simulink model "PPS_Scenario_006_cs"  (Simulink 7.6)
settings: Solver=ode5  SolverMode=SingleTasking  StartTime=0.0  StopTime=inf  FixedStep=1/100  RelTol=1e-3
PreLoadFcn:
  | check_NUTS_defined;
  | 
  | assignin('base',['model_closed_' bdroot],false);
  | 
  | addpath('../includes_PPS');
  | 
  | if exist('PPS_Model_sfun.mexw64')==3
  | delete PPS_Model_sfun.mexw64;
  | end
  | 
  | if exist('PPS_Model_sfun.mexw32') ==3
  | delete PPS_Model_sfun.mexw32;
  | end
  | 
  | switch version('-release')
  | case {'2010a', '2010b', '2011a'}
  | addpath('../includes_PPS/ML2010a');
  | case {'2011b', '2012a', '2012b'}
  | addpath('../includes_PPS/ML2011b');
  | otherwise
  | addpath('../includes_PPS/ML2011b');
  | end
InitFcn:
  | PreScanExperimentInitFcn(bdroot)
StopFcn:
  | PreScanExperimentStopFcn(bdroot)
undefined symbols (not defined in the file): DiscIntNeverNeededParam, InitImageOutputDir, x_ini_VRML, y_ini_VRML, z_ini_VRML
libraries: PreScanSimulinkLibrary x48, simulink x27, PreScanUsefulBlocks x20, simulink_extras x9, simulink_need_slupdate x1
(part 10 of 14)

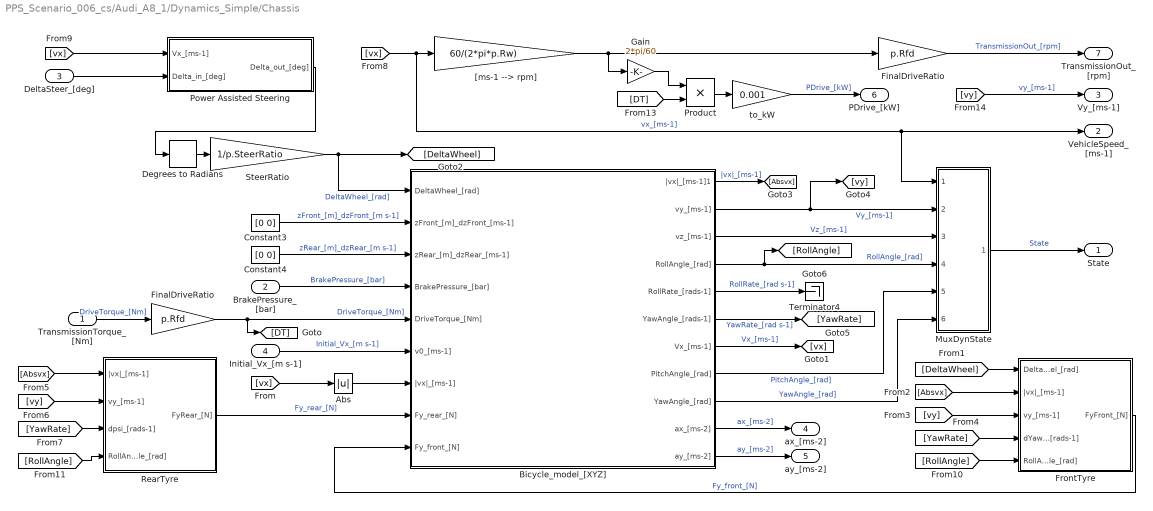
== system PPS_Scenario_006_cs/Audi_A8_1/Dynamics_Simple/Chassis ==
  TransmissionTorque_[Nm] : Inport
  BrakePressure_[bar] : Inport  Port=2
  DeltaSteer_[deg] : Inport  Port=3
  Initial_Vx_[m s-1] : Inport  Port=4
  Abs : Abs
  Bicycle_model_[XYZ] : Subsystem
      mask Display: image(imread('Bicycle_model.png'));
  Constant3 : Constant  Value=[0 0]
  Constant4 : Constant  Value=[0 0]
  Degrees to Radians : simulink_extras/Transformations/Degrees to Radians  SystemSampleTime=-1
  FinalDriveRatio : Gain  Gain=p.Rfd  SaturateOnIntegerOverflow=on  OutDataTypeStr=Inherit: Same as input  ParamDataTypeStr=Inherit: Same as input
  "FinalDriveRatio " : Gain  Gain=p.Rfd  SaturateOnIntegerOverflow=on  OutDataTypeStr=Inherit: Same as input  ParamDataTypeStr=Inherit: Same as input
  FrontTyre : Subsystem
      mask Display: image(imread('Tyre.png'));
  Gain : Gain  Gain=2*pi/60
  MuxDynState : Subsystem
  Power Assisted Steering : Subsystem
  Product : Product  RndMeth=Zero
  RearTyre : Subsystem
      mask Display: image(imread('Tyre.png'));
  SteerRatio : Gain  Gain=1/p.SteerRatio
  Terminator4 : Terminator
  "[ms-1 --> rpm]" : Gain  Gain=60/(2*pi*p.Rw)  SaturateOnIntegerOverflow=on  OutDataTypeStr=Inherit: Same as input  ParamDataTypeStr=Inherit: Same as input
  to_kW : Gain  Gain=0.001
  State : Outport
  VehicleSpeed_[ms-1] : Outport  Port=2
  Vy_[ms-1] : Outport  Port=3
  ax_[ms-2] : Outport  Port=4
  ay_[ms-2] : Outport  Port=5
  PDrive_[kW] : Outport  Port=6
  TransmissionOut_[rpm] : Outport  Port=7
  wires:
  [vy] -> Vy_[ms-1]/1  "vy_[ms-1]"
  to_kW/1 -> PDrive_[kW]/1  "PDrive_[kW]"
  Gain/1 -> Product/1
  Bicycle_model_[XYZ]/10(ax_[ms-2]) -> ax_[ms-2]/1  "ax_[ms-2]"
  Product/1 -> to_kW/1
  [DT] -> Product/2
  Bicycle_model_[XYZ]/11(ay_[ms-2]) -> ay_[ms-2]/1  "ay_[ms-2]"
  Abs/1 -> Bicycle_model_[XYZ]/7(|vx|_[ms-1])
  Degrees to Radians/1 -> SteerRatio/1
  [vx] -> Abs/1
  SteerRatio/1 -> [DeltaWheel], Bicycle_model_[XYZ]/1(DeltaWheel_[rad])  "DeltaWheel_[rad]"
  TransmissionTorque_[Nm]/1 -> "FinalDriveRatio "/1  "DriveTorque_[Nm]"
  RearTyre/1(FyRear_[N]) -> Bicycle_model_[XYZ]/8(Fy_rear_[N])  "Fy_rear_[N]"
  FrontTyre/1(FyFront_[N]) -> Bicycle_model_[XYZ]/9(Fy_front_[N])  "Fy_front_[N]"
  Bicycle_model_[XYZ]/1(|vx|_[ms-1]1) -> [Absvx]  "|vx|_[ms-1]"
  Bicycle_model_[XYZ]/2(vy_[ms-1]) -> [vy], MuxDynState/2(vy [ms-1])  "Vy_[ms-1]"
  Bicycle_model_[XYZ]/4(RollAngle_[rad]) -> MuxDynState/4(R [rad]), [RollAngle]  "RollAngle_[rad]"
  Bicycle_model_[XYZ]/6(YawAngle_[rads-1]) -> [YawRate]  "YawRate_[rad s-1]"
  Bicycle_model_[XYZ]/7(Vx_[ms-1]) -> [vx]  "Vx_[ms-1]"
  [DeltaWheel] -> FrontTyre/1(DeltaWheel_[rad])
  [Absvx] -> FrontTyre/2(|vx|_[ms-1])
  [vy] -> FrontTyre/3(vy_[ms-1])
  [YawRate] -> FrontTyre/4(dYawAngle_[rads-1])
  [Absvx] -> RearTyre/1(|vx|_[ms-1])
  [vy] -> RearTyre/2(vy_[ms-1])
  [YawRate] -> RearTyre/3(dpsi_[rads-1])
  Bicycle_model_[XYZ]/3(vz_[ms-1]) -> MuxDynState/3(vz [ms-1])  "Vz_[ms-1]"
  Bicycle_model_[XYZ]/8(PitchAngle_[rad]) -> MuxDynState/5(P [rad])  "PitchAngle_[rad]"
  Bicycle_model_[XYZ]/9(YawAngle_[rad]) -> MuxDynState/6(Y [rad])  "YawAngle_[rad]"
  "[ms-1 --> rpm]"/1 -> Gain/1, FinalDriveRatio/1
  FinalDriveRatio/1 -> TransmissionOut_[rpm]/1  "TransmissionOut_[rpm]"
  [vx] -> "[ms-1 --> rpm]"/1, VehicleSpeed_[ms-1]/1, MuxDynState/1(vx [ms-1])  "vx_[ms-1]"
  [vx] -> Power Assisted Steering/1(Vx_[ms-1])
  DeltaSteer_[deg]/1 -> Power Assisted Steering/2(Delta_in_[deg])
  Power Assisted Steering/1(Delta_out_[deg]) -> Degrees to Radians/1
  [RollAngle] -> FrontTyre/5(RollAngle_[rad])
  [RollAngle] -> RearTyre/4(RollAngle_[rad])
  Constant3/1 -> Bicycle_model_[XYZ]/2(zFront_[m]_dzFront_[ms-1])  "zFront_[m]_dzFront_[m s-1]"
  Constant4/1 -> Bicycle_model_[XYZ]/3(zRear_[m]_dzRear_[ms-1])  "zRear_[m]_dzRear_[m s-1]"
  BrakePressure_[bar]/1 -> Bicycle_model_[XYZ]/4(BrakePressure_[bar])  "BrakePressure_[bar]"
  "FinalDriveRatio "/1 -> Bicycle_model_[XYZ]/5(DriveTorque_[Nm]), [DT]  "DriveTorque_[Nm]"
  Initial_Vx_[m s-1]/1 -> Bicycle_model_[XYZ]/6(v0_[ms-1])  "Initial_Vx_[m s-1]"
  Bicycle_model_[XYZ]/5(RollRate_[rads-1]) -> Terminator4/1  "RollRate_[rad s-1]"
  MuxDynState/1(State) -> State/1  "State"

== system PPS_Scenario_006_cs/Audi_A8_1/Dynamics_Simple/Engine ==
  ImpellerTorque_[Nm] : Inport
  Throttle_[%] : Inport  Port=2
  Configurable Subsystem : Subsystem  BlockChoice=Discrete Rate Limiter  mask{ComputationMode=ComputationMode}
      mask prompts: ComputationMode "Compuation mode:"
      mask init:
      | SetComputationMode(gcb,ComputationMode);
      settings: AttributesFormatString=%<BlockChoice>  OpenFcn=BringToFront(gcb);  MemberBlocks=Discrete Rate Limiter,Rate Limiter
      settings: TemplateBlock=|
      | PreScanSimulinkLibrary/Configurable Subsystems/TransferFunction
      | Engine/Configurable
      | Subsystem
  Configurable Subsystem1 : Subsystem  BlockChoice=Discrete-Time Integrator  mask{ComputationMode=ComputationMode}
      mask prompts: ComputationMode "Computation mode:"
      mask init:
      | SetComputationMode(gcb,ComputationMode);
      settings: AttributesFormatString=%<BlockChoice>  OpenFcn=BringToFront(gcb);  MemberBlocks=Discrete-Time Integrator,Integrator
      settings: TemplateBlock=|
      | PreScanSimulinkLibrary/Configurable Subsystems/integral with initial condition and limts
      | for engine/Configurable
      | Subsystem
  EngineTorque : Lookup2D  RowIndex=p.thvec  ColumnIndex=p.nevec  Table=p.emap  InputSameDT=on
  Gain : Gain  Gain=2*pi/60
  Product : Product  RndMeth=Zero
  Sum : Sum  Inputs=-+  SaturateOnIntegerOverflow=on  InputSameDT=on  OutDataTypeStr=Inherit: Same as first input
  engine + impeller inertia : Gain  Gain=1/p.Iei  SaturateOnIntegerOverflow=on  OutDataTypeStr=Inherit: Same as input  ParamDataTypeStr=Inherit: Same as input
  to_kW : Gain  Gain=0.001
  nEngine_[rpm] : Outport  InitialOutput=0
  PEngine_[kW] : Outport  Port=2  InitialOutput=0
  wires:
  EngineTorque/1 -> Sum/2, Product/2
  engine + impeller inertia/1 -> Configurable Subsystem1/1(In1)
  Sum/1 -> engine + impeller inertia/1
  Configurable Subsystem1/1(Out1) -> nEngine_[rpm]/1, EngineTorque/2, Gain/1  "rpm"
  Throttle_[%]/1 -> Configurable Subsystem/1(In1)
  ImpellerTorque_[Nm]/1 -> Sum/1
  Configurable Subsystem/1(Out1) -> EngineTorque/1
  Product/1 -> to_kW/1
  Gain/1 -> Product/1
  to_kW/1 -> PEngine_[kW]/1

== system PPS_Scenario_006_cs/Audi_A8_1/Dynamics_Simple/Gear: Auto Manual ==
  note: 0; Auto = on // Manual =off
      | 1; Auto = off // Manual =on
  Auto_Manual : Inport
  Manual_Gear : Inport  Port=2
  Auto_Gear : Inport  Port=3
  If : If  IfExpression=u1 == 0
  If Action Subsystem : Subsystem  TreatAsAtomicUnit=on
  If Action Subsystem1 : Subsystem  TreatAsAtomicUnit=on
  Merge : Merge
  Gear : Outport
  wires:
  If Action Subsystem/1(Out1) -> Merge/1
  Auto_Gear/1 -> If Action Subsystem/1(In1)
  If/1 -> If Action Subsystem/Action
  Merge/1 -> Gear/1
  If Action Subsystem1/1(Out1) -> Merge/2
  Manual_Gear/1 -> If Action Subsystem1/1(In1)
  If/2 -> If Action Subsystem1/Action
  Auto_Manual/1 -> If/1

== system PPS_Scenario_006_cs/Audi_A8_1/Dynamics_Simple/ShiftLogic ==
  Throttle_[%] : Inport
  GearNr_[-] : Inport  Port=2
  Auto_GearShift : Inport  Port=3
  VehSpeed_[ms-1] : Inport  Port=4
  Add2 : Sum
  Data Type Conversion1 : DataTypeConversion  OutDataTypeStr=double
  Detect Increase1 : simulink/Logic and Bit Operations/Detect Increase  SystemSampleTime=-1  vinit=0.0
  Detect Increase : Subsystem
  Gear limitation : Saturate  UpperLimit=p.maxGear  LowerLimit=1
  Gear limitation while shifting : Saturate  UpperLimit=p.maxGear  LowerLimit=1
  GearNeutral : Constant  Value=0
  GearReverse : Constant  Value=-1
  "IC, gear = 1" : Memory  X0=1  InheritSampleTime=on
  If Action Neutral : Subsystem  TreatAsAtomicUnit=on
  If Action Normal : Subsystem  TreatAsAtomicUnit=on
  If Action Reverse : Subsystem  TreatAsAtomicUnit=on
  Memory : Memory  InheritSampleTime=on
  Merge : Merge  Inputs=3
  Relational Operator : RelationalOperator  OutDataTypeStr=boolean
  Relational Operator1 : RelationalOperator  Operator=<=  OutDataTypeStr=boolean
  Shift_Down time : simulink/Discrete/Integer Delay  NumDelays=p.ShiftDown_fac  InputProcessing=Inherited  vinit=0.0  samptime=-1
  Shift_Up time : simulink/Discrete/Integer Delay  NumDelays=p.ShiftUp_fac  InputProcessing=Inherited  vinit=0.0  samptime=-1
  Sum : Sum  Inputs=+-
  interp_down : Lookup2D  RowIndex=p.downth  ColumnIndex=[1:p.maxGear]  Table=p.downtab  LookUpMeth=Interpolation-Use End Values  InputSameDT=on
  interp_up : Lookup2D  RowIndex=p.upth  ColumnIndex=[1:p.maxGear]  Table=p.uptab  LookUpMeth=Interpolation-Use End Values  InputSameDT=on
  reverse/neutral/normal gear : If  IfExpression=u1 == 0  ElseIfExpressions=u1 < 0
  to_ms-1 : Gain  Gain=1/3.6
  "to_ms-1 " : Gain  Gain=1/3.6
  GearNr : Outport
  wires:
  Auto_GearShift/1 -> reverse/neutral/normal gear/1
  "IC, gear = 1"/1 -> If Action Normal/1(In1)
  Merge/1 -> GearNr/1
  If Action Reverse/1(Out1) -> Merge/2
  If Action Neutral/1(Out1) -> Merge/1
  If Action Normal/1(Out1) -> Merge/3
  reverse/neutral/normal gear/3 -> If Action Normal/Action
  reverse/neutral/normal gear/1 -> If Action Neutral/Action
  reverse/neutral/normal gear/2 -> If Action Reverse/Action
  GearReverse/1 -> If Action Reverse/1(In1)
  GearNeutral/1 -> If Action Neutral/1(In1)
  Shift_Down time/1 -> Sum/2
  Shift_Up time/1 -> Sum/1
  Detect Increase/1(Out1) -> Shift_Up time/1
  Data Type Conversion1/1 -> Shift_Down time/1
  Detect Increase1/1 -> Data Type Conversion1/1
  Sum/1 -> Add2/1
  Memory/1 -> Add2/2  "GearNr_[-]"
  Add2/1 -> Gear limitation while shifting/1
  Gear limitation while shifting/1 -> "IC, gear = 1"/1, Memory/1  "GearNr_[-]"
  Throttle_[%]/1 -> interp_down/1, interp_up/1
  Relational Operator/1 -> Detect Increase/2(In2)
  Relational Operator1/1 -> Detect Increase1/1
  interp_down/1 -> "to_ms-1 "/1
  VehSpeed_[ms-1]/1 -> Relational Operator/1, Relational Operator1/1
  interp_up/1 -> to_ms-1/1
  Gear limitation/1 -> interp_down/2, interp_up/2, Detect Increase/1(GearNr_[-])
  GearNr_[-]/1 -> Gear limitation/1
  to_ms-1/1 -> Relational Operator/2
  "to_ms-1 "/1 -> Relational Operator1/2

== system PPS_Scenario_006_cs/Audi_A8_1/Dynamics_Simple/Transmission ==
  nEngine_[rpm] : Inport
  GearNr_[-] : Inport  Port=2
  n_TransmissionOut_[rpm] : Inport  Port=3
  Torque_Converter : Subsystem
      mask Display: image(imread('TorqueConverter.png'));
  Transmission_Ratio : Subsystem
  Viscous coupling : Lookup  InputValues=[-5:0.1:5]*p.m/4  Table=p.m/4*tanh([-5:0.1:5])
  ImpellerTorque_[Nm] : Outport  InitialOutput=0
  TransmissionTorque_[Nm] : Outport  Port=2  InitialOutput=0
  wires:
  Torque_Converter/2(TurbineTorque_[Nm]) -> Viscous coupling/1  "Converter_Torque_[Nm]"
  Transmission_Ratio/2(nTransmissionIn_[rpm]) -> Torque_Converter/2(nTransmission_[rpm])
  nEngine_[rpm]/1 -> Torque_Converter/1(nEngine_[rpm])
  GearNr_[-]/1 -> Transmission_Ratio/2(GearNr_[-]), Torque_Converter/3(Gear nr)
  n_TransmissionOut_[rpm]/1 -> Transmission_Ratio/3(nTransmissionOut_[rpm])
  Torque_Converter/1(ImpellerTorque_[Nm]) -> ImpellerTorque_[Nm]/1
  Transmission_Ratio/1(tTransmissionOut_[Nm]) -> TransmissionTorque_[Nm]/1
  Viscous coupling/1 -> Transmission_Ratio/1(tTransmissionIn_[Nm])

== system PPS_Scenario_006_cs/Audi_A8_1/PathFollower_1/CTRL REFERENCES ==
  note: REFERENCE POSITION BASED POSITION CTRL
  Pos x,y,Y [m,m,rad] : Inport
  Position Preview Distance [m] : Inport  Port=2
  TrajOffset [m,m,rad] : Inport  Port=3
  ActorOffset_Left(+) / Right(-)_[m] : Inport  Port=4
  Calculate Preview Point (pvp) by extrapolating current Vehicle Position (p0) with Preview Distance and Vehicle Orientation : Subsystem
  Find Reference Point (pref)  on Trajectory closest  to PreView Point (pvp) : M-S-Function  FunctionName=msfcn_find_closest_trajectory_points  Parameters=[Traj_x Traj_y]
      mask Display:
      | port_label('input', 1, 'pvp')
      | port_label('input', 2, 'TrajOffset_x_y_Y')
      | port_label('input', 3, 'ActorOffset_Left+/Right-')
      | port_label('input', 4, 'p0')
      | port_label('output', 1, 'pref')
  Find Reference Point (pref0)  on Trajectory closest  to P0 Point (p0) : M-S-Function  FunctionName=msfcn_find_closest_trajectory_points0  Parameters=[Traj_x Traj_y]
      mask Display:
      | port_label('input', 1, 'pvp')
      | port_label('input', 2, 'TrajOffset_x_y_Y')
      | port_label('input', 3, 'ActorOffset_Left+/Right-')
      | port_label('input', 4, 'p0')
      | port_label('output', 1, 'pref_0')
      | port_label('output', 2, 'Actor/Traj_distance')
      | port_label('output', 3, 'Actor/Traj_angle')
  Mux1 : Mux  Inputs=2
  Selector1 : Selector  InputPortWidth=3  IndexOptions=Index vector (dialog)  Indices=[1 2]  OutputSizes=1
  Terminator : Terminator
  pvp  [m,m] : Outport
  pref_pvp [m,m] : Outport  Port=2
  pref_0 [m,m] : Outport  Port=3
  Actor/Traj_distance [m] : Outport  Port=4
  Actor/Traj_angle [deg] : Outport  Port=5
  wires:
  Mux1/1 -> pvp  [m,m]/1, Find Reference Point (pref)  on Trajectory closest  to PreView Point (pvp)/1, Find Reference Point (pref0)  on Trajectory closest  to P0 Point (p0)/1
  Pos x,y,Y [m,m,rad]/1 -> Calculate Preview Point (pvp) by extrapolating current Vehicle Position (p0) with Preview Distance and Vehicle Orientation/2(x,y,Y Demux [m,m,rad]), Find Reference Point (pref0)  on Trajectory closest  to P0 Point (p0)/4, Selector1/1
  Calculate Preview Point (pvp) by extrapolating current Vehicle Position (p0) with Preview Distance and Vehicle Orientation/1(x_glob_PVD) -> Mux1/1
  Calculate Preview Point (pvp) by extrapolating current Vehicle Position (p0) with Preview Distance and Vehicle Orientation/3(Y [rad]) -> Terminator/1
  Position Preview Distance [m]/1 -> Calculate Preview Point (pvp) by extrapolating current Vehicle Position (p0) with Preview Distance and Vehicle Orientation/1(Preview Distance)
  Find Reference Point (pref)  on Trajectory closest  to PreView Point (pvp)/1 -> pref_pvp [m,m]/1
  Find Reference Point (pref0)  on Trajectory closest  to P0 Point (p0)/1 -> pref_0 [m,m]/1
  Calculate Preview Point (pvp) by extrapolating current Vehicle Position (p0) with Preview Distance and Vehicle Orientation/2(y_glob_PVD) -> Mux1/2
  TrajOffset [m,m,rad]/1 -> Find Reference Point (pref)  on Trajectory closest  to PreView Point (pvp)/2, Find Reference Point (pref0)  on Trajectory closest  to P0 Point (p0)/2  "L6"
  ActorOffset_Left(+) / Right(-)_[m]/1 -> Find Reference Point (pref)  on Trajectory closest  to PreView Point (pvp)/3, Find Reference Point (pref0)  on Trajectory closest  to P0 Point (p0)/3
  Selector1/1 -> Find Reference Point (pref)  on Trajectory closest  to PreView Point (pvp)/4
  Find Reference Point (pref0)  on Trajectory closest  to P0 Point (p0)/2 -> Actor/Traj_distance [m]/1
  Find Reference Point (pref0)  on Trajectory closest  to P0 Point (p0)/3 -> Actor/Traj_angle [deg]/1

== system PPS_Scenario_006_cs/Audi_A8_1/PathFollower_1/Calculate shifted p0 wrt COG ==
  position x,y,Y [m,m,deg] : Inport
  Constant1 : Constant  Value=XShifting_wrt_COG
  Degrees to Radians : simulink_extras/Transformations/Degrees to Radians  SystemSampleTime=-1
  Demux1 : Demux  Outputs=3
  Fcn : Fcn  Expr=u(2)*cos(u(1))
  Fcn1 : Fcn  Expr=u(2)*sin(u(1))
  Mux1 : Mux  Inputs=3
  Mux2 : Mux  Inputs=2
  Sum : Sum  Inputs=|++
  Sum1 : Sum  Inputs=|++
  position x,y,Y [m,m,rad] : Outport
  wires:
  Sum/1 -> Mux1/1
  Sum1/1 -> Mux1/2
  Demux1/1 -> Sum/1
  Demux1/3 -> Degrees to Radians/1
  Degrees to Radians/1 -> Mux2/1, Mux1/3
  Mux2/1 -> Fcn/1, Fcn1/1
  Fcn/1 -> Sum/2
  Fcn1/1 -> Sum1/2
  Demux1/2 -> Sum1/1
  position x,y,Y [m,m,deg]/1 -> Demux1/1
  Mux1/1 -> position x,y,Y [m,m,rad]/1
  Constant1/1 -> Mux2/2

== system PPS_Scenario_006_cs/Audi_A8_1/PathFollower_1/DELTA CTRL ==
  note: POSITION BASED STEERWHEEL CONTROL
  p0 : Inport
  pvp : Inport  Port=2
  pref_pvp : Inport  Port=3
  pref0 : Inport  Port=4
  Calculate  preview angle : M-S-Function  FunctionName=msfcn_preview_angle_and_distance
      mask Display:
      | port_label('input', 2, 'pref [m,m]')
      | port_label('input', 3, 'p0 [m,m]')
      | port_label('input', 1, 'pvp [m,m]')
      | 
      | port_label('output', 1, 'angle [rad]')
  Divide2 : Product
  Divide4 : Product
  Error check : Subsystem
  Goto Tag Visibility : GotoTagVisibility  GotoTag=pref0
  Goto Tag Visibility1 : GotoTagVisibility  GotoTag=p0
  Radians to Degrees1 : simulink_extras/Transformations/Radians to Degrees  SystemSampleTime=-1
  Selector2 : Selector  InputPortWidth=3  IndexOptions=Index vector (dialog)  Indices=[1 2]  OutputSizes=1
  Steering angle  velocity dependent : Lookup  InputValues=[0 18 40 60 70 80 90 100 110]  Table=[16.5 16.5 28 44.5 55 60.5 60.5 60.5 60.5]
  Steering angle preview  distance dependent : Lookup  InputValues=[0 1 4 5 6 7 8 9 10 11 20 21]  Table=[1.5 1.5 1 1 1 1 1 1 0.9 0.9 0.8 0.8]
  These limits are  the vehicle maximum  steering wheel angle : Saturate  UpperLimit=720  LowerLimit=-720
  TunableSteering Gain : Gain  Gain=TunableSteeringGain
  sign1 : Gain  Gain=3.6
  delta_steerwheel [deg] : Outport
  tag scope: p0=scoped, pref0=scoped
  wires:
  Calculate  preview angle/1 -> Radians to Degrees1/1
  Selector2/1 -> Calculate  preview angle/3
  p0/1 -> Selector2/1, [p0]
  pvp/1 -> Calculate  preview angle/1
  pref_pvp/1 -> Calculate  preview angle/2
  Radians to Degrees1/1 -> Divide2/2
  These limits are  the vehicle maximum  steering wheel angle/1 -> delta_steerwheel [deg]/1
  pref0/1 -> [pref0]
  sign1/1 -> Steering angle  velocity dependent/1
  [v_actual] -> sign1/1
  Steering angle  velocity dependent/1 -> Divide2/1
  Divide4/1 -> TunableSteering Gain/1
  Divide2/1 -> Divide4/1
  Steering angle preview  distance dependent/1 -> Divide4/2
  [PreviewDistance] -> Steering angle preview  distance dependent/1
  TunableSteering Gain/1 -> These limits are  the vehicle maximum  steering wheel angle/1

== system PPS_Scenario_006_cs/Audi_A8_1/PathFollower_1/THROTTLE CTRL ==
  v_actual [m/s] : Inport
  Desired Velocity [m/s] : Inport  Port=2
  Initial Velocity [m/s] : Inport  Port=3
  Demux : Demux  Outputs=3
  GearNormal : Constant
  "GearNormal " : Constant
  If Desired Velocity = 0 : Subsystem  TreatAsAtomicUnit=on
  If Desired Velocity ~= 0 : Subsystem  TreatAsAtomicUnit=on
  Merge : Merge
  Mux : Mux  Inputs=3
  Mux2 : Mux  Inputs=3
  Sum4 : Sum  Inputs=|+-
  if : If  IfExpression=u1 == 0
  throttle [%] : Outport
  brake pressure [bar] : Outport  Port=2
  v0 [m/s] : Outport  Port=3
  Auto_GearShift : Outport  Port=4
  wires:
  v_actual [m/s]/1 -> Sum4/2
  If Desired Velocity ~= 0/3(Auto_GearShift) -> Mux2/3
  If Desired Velocity ~= 0/2(brake pressure [bar]) -> Mux2/2
  If Desired Velocity ~= 0/1(throttle [%]) -> Mux2/1
  if/1 -> If Desired Velocity = 0/Action
  if/2 -> If Desired Velocity ~= 0/Action
  If Desired Velocity = 0/3(Auto_GearShift) -> Mux/3
  "GearNormal "/1 -> If Desired Velocity ~= 0/1(In1)
  Demux/3 -> Auto_GearShift/1
  Demux/2 -> brake pressure [bar]/1
  Demux/1 -> throttle [%]/1
  Mux/1 -> Merge/1
  Mux2/1 -> Merge/2
  If Desired Velocity = 0/2(brake pressure [bar]) -> Mux/2
  If Desired Velocity = 0/1(throttle [%]) -> Mux/1
  Merge/1 -> Demux/1
  GearNormal/1 -> If Desired Velocity = 0/1(In1)
  Initial Velocity [m/s]/1 -> v0 [m/s]/1
  Desired Velocity [m/s]/1 -> Sum4/1, if/1
  Sum4/1 -> If Desired Velocity ~= 0/2(Desired Velocity [m/s])

== system PPS_Scenario_006_cs/Audi_A8_1/SELF_Demux/compas converter ==
  rotz [rad] : Inport
  cart2compas : Subsystem
  rad2deg : Gain  Gain=180/pi
  heading [deg] : Outport
  wires:
  cart2compas/1(heading [deg]) -> heading [deg]/1
  rotz [rad]/1 -> rad2deg/1
  rad2deg/1 -> cart2compas/1(Angle [deg])

== system PPS_Scenario_006_cs/Audi_A8_1/Trajectories/Car_trajectory_1 ==
  From Workspace : FromWorkspace  VariableName=trajectory  SampleTime=TimeStep  OutputAfterFinalValue=Holding final value
  From Workspace1 : FromWorkspace  VariableName=trajectory  SampleTime=TimeStep  OutputAfterFinalValue=Setting to zero
  Mux : Mux  Inputs=2
  Selector1 : Selector  InputPortWidth=24  IndexOptions=Index vector (dialog)  Indices=[7:18]  OutputSizes=1
  Selector9 : Selector  InputPortWidth=24  IndexOptions=Index vector (dialog)  Indices=[1:6]  OutputSizes=1
  trajectory : Outport
  wires:
  Selector1/1 -> Mux/2
  Selector9/1 -> Mux/1
  Mux/1 -> trajectory/1
  From Workspace1/1 -> Selector1/1
  From Workspace/1 -> Selector9/1

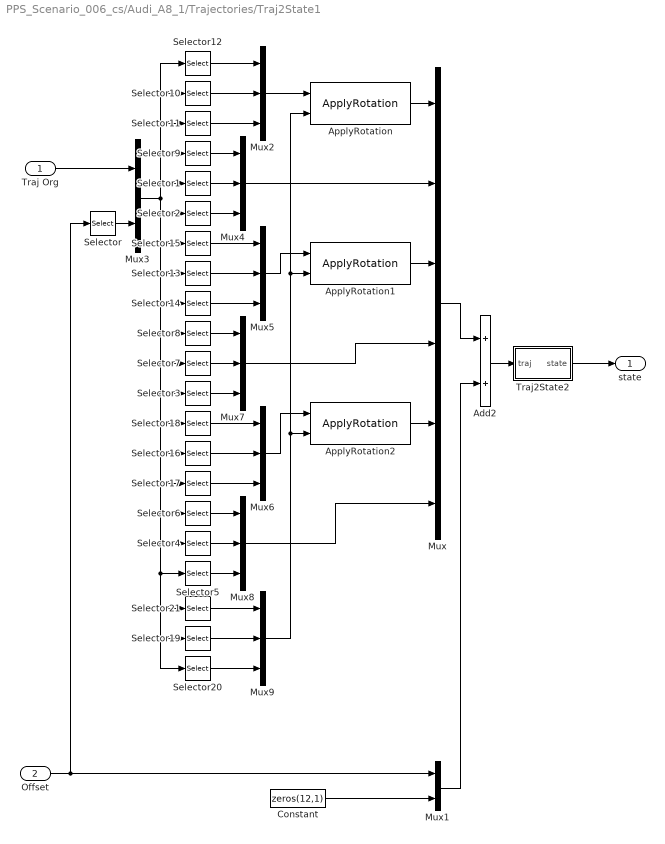
== system PPS_Scenario_006_cs/Audi_A8_1/Trajectories/Traj2State1 ==
  Traj Org : Inport
  Offset : Inport  Port=2
  Add2 : Sum
  ApplyRotation : PreScanSimulinkLibrary/ApplyRotation  SystemSampleTime=-1
  ApplyRotation1 : PreScanSimulinkLibrary/ApplyRotation  SystemSampleTime=-1
  ApplyRotation2 : PreScanSimulinkLibrary/ApplyRotation  SystemSampleTime=-1
  Constant : Constant  Value=zeros(12,1)
  Mux : Mux  Inputs=6
  Mux1 : Mux  Inputs=2
  Mux{2,4..9} (7 alike) : Mux  Inputs=3
  Mux3 : Mux  Inputs=2
  Selector : Selector  InputPortWidth=6  IndexOptions=Index vector (dialog)  Indices=[4 5 6]  OutputSizes=1
  Selector1 : Selector  InputPortWidth=21  IndexOptions=Index vector (dialog)  Indices=[5]  OutputSizes=1
  Selector10 : Selector  InputPortWidth=21  IndexOptions=Index vector (dialog)  Indices=[2]  OutputSizes=1
  Selector11 : Selector  InputPortWidth=21  IndexOptions=Index vector (dialog)  Indices=[3]  OutputSizes=1
  Selector12 : Selector  InputPortWidth=21  IndexOptions=Index vector (dialog)  Indices=[1]  OutputSizes=1
  Selector13 : Selector  InputPortWidth=21  IndexOptions=Index vector (dialog)  Indices=[8]  OutputSizes=1
  Selector14 : Selector  InputPortWidth=21  IndexOptions=Index vector (dialog)  Indices=[9]  OutputSizes=1
  Selector15 : Selector  InputPortWidth=21  IndexOptions=Index vector (dialog)  Indices=[7]  OutputSizes=1
  Selector16 : Selector  InputPortWidth=21  IndexOptions=Index vector (dialog)  Indices=[14]  OutputSizes=1
  Selector17 : Selector  InputPortWidth=21  IndexOptions=Index vector (dialog)  Indices=[15]  OutputSizes=1
  Selector18 : Selector  InputPortWidth=21  IndexOptions=Index vector (dialog)  Indices=[13]  OutputSizes=1
  Selector19 : Selector  InputPortWidth=21  IndexOptions=Index vector (dialog)  Indices=[20]  OutputSizes=1
  Selector2 : Selector  InputPortWidth=21  IndexOptions=Index vector (dialog)  Indices=[6]  OutputSizes=1
  Selector20 : Selector  InputPortWidth=21  IndexOptions=Index vector (dialog)  Indices=[21]  OutputSizes=1
  Selector21 : Selector  InputPortWidth=21  IndexOptions=Index vector (dialog)  Indices=[19]  OutputSizes=1
  Selector3 : Selector  InputPortWidth=21  IndexOptions=Index vector (dialog)  Indices=[12]  OutputSizes=1
  Selector4 : Selector  InputPortWidth=21  IndexOptions=Index vector (dialog)  Indices=[17]  OutputSizes=1
  Selector5 : Selector  InputPortWidth=21  IndexOptions=Index vector (dialog)  Indices=[18]  OutputSizes=1
  Selector6 : Selector  InputPortWidth=21  IndexOptions=Index vector (dialog)  Indices=[16]  OutputSizes=1
  Selector7 : Selector  InputPortWidth=21  IndexOptions=Index vector (dialog)  Indices=[11]  OutputSizes=1
  Selector8 : Selector  InputPortWidth=21  IndexOptions=Index vector (dialog)  Indices=[10]  OutputSizes=1
  Selector9 : Selector  InputPortWidth=21  IndexOptions=Index vector (dialog)  Indices=[4]  OutputSizes=1
  Traj2State2 : Subsystem
  state : Outport
  wires:
  Mux9/1 -> ApplyRotation2/2, ApplyRotation1/2, ApplyRotation/2
  Selector20/1 -> Mux9/3
  Selector19/1 -> Mux9/2
  Selector21/1 -> Mux9/1
  Selector5/1 -> Mux8/3
  Selector4/1 -> Mux8/2
  Selector6/1 -> Mux8/1
  Mux8/1 -> Mux/6
  Mux6/1 -> ApplyRotation2/1
  Mux7/1 -> Mux/4
  ApplyRotation2/1 -> Mux/5
  Selector3/1 -> Mux7/3
  Selector7/1 -> Mux7/2
  Selector8/1 -> Mux7/1
  Mux4/1 -> Mux/2
  Mux5/1 -> ApplyRotation1/1
  ApplyRotation1/1 -> Mux/3
  Mux2/1 -> ApplyRotation/1
  ApplyRotation/1 -> Mux/1
  Selector2/1 -> Mux4/3
  Selector1/1 -> Mux4/2
  Selector9/1 -> Mux4/1
  Selector17/1 -> Mux6/3
  Selector16/1 -> Mux6/2
  Selector18/1 -> Mux6/1
  Selector14/1 -> Mux5/3
  Selector13/1 -> Mux5/2
  Selector15/1 -> Mux5/1
  Selector11/1 -> Mux2/3
  Selector10/1 -> Mux2/2
  Selector12/1 -> Mux2/1
  Mux3/1 -> Selector8/1, Selector7/1, Selector3/1, Selector18/1, Selector16/1, Selector17/1, Selector6/1, Selector20/1, Selector19/1, Selector21/1, Selector5/1, Selector4/1, Selector14/1, Selector13/1, Selector15/1, Selector2/1, Selector1/1, Selector9/1, Selector12/1, Selector10/1, Selector11/1
  Mux1/1 -> Add2/2
  Constant/1 -> Mux1/2
  Add2/1 -> Traj2State2/1(traj)
  Selector/1 -> Mux3/2
  Traj Org/1 -> Mux3/1
  Offset/1 -> Mux1/1, Selector/1
  Mux/1 -> Add2/1
  Traj2State2/1(state) -> state/1

== system PPS_Scenario_006_cs/BMW_X5_1/Dynamics_Empty/MuxState ==
  note: mode: Dynamics
  note: mode: Positioning
  note: mode: Dynamics
      | VelVEHICLE
      | wrt VEH
  note: AnglesVEHICLE
      | wrtGLOB
  note: For state mode 'Dynamic' positions
      | are not taken into account, as they
      | are computed by integrating velocity.
      | Click annotation for Help.
  x [m] : Inport  SampleTime=TimeStep
  y [m] : Inport  Port=2  SampleTime=TimeStep
  z [m] : Inport  Port=3  SampleTime=TimeStep
  dx [m/s] : Inport  Port=4  SampleTime=TimeStep
  dy [m/s] : Inport  Port=5  SampleTime=TimeStep
  dz [m/s] : Inport  Port=6  SampleTime=TimeStep
  R [rad] : Inport  Port=7  SampleTime=TimeStep
  P [rad] : Inport  Port=8  SampleTime=TimeStep
  Y [rad] : Inport  Port=9  SampleTime=TimeStep
  Constant : Constant  DisableCoverage=on  Value=positioningmode
  Discrete-Time Integrator : DiscreteIntegrator  SampleTime=TimeStep  ICPrevOutput=DiscIntNeverNeededParam  ICPrevScaledInput=DiscIntNeverNeededParam
  Ground : Ground
  Ground1 : Ground
  Mux1 : Mux  Inputs=[3 3]
  Mux2 : Mux  Inputs=3
  Mux3 : Mux  Inputs=3
  Mux4 : Mux  Inputs=3
  Mux5 : Mux  Inputs=[3 3]
  Mux6 : Mux  Inputs=[6 3]
  Switch : Switch  Threshold=0.5
  Transformation_BODY2GLOBAL : PreScanSimulinkLibrary/Simple_Vehicle_Dynamics/Chassis/MuxDynState/Transformation_BODY2GLOBAL  SystemSampleTime=-1
  mux3 : Mux  Inputs=3
  state : Outport
  wires:
  Constant/1 -> Switch/2
  Mux6/1 -> state/1
  Mux4/1 -> Mux1/1
  Mux5/1 -> Switch/3
  Mux1/1 -> Switch/1
  Switch/1 -> Mux6/1  "PosVeh wrt  GLOB"
  P [rad]/1 -> Mux3/2
  R [rad]/1 -> Mux3/1
  dz [m/s]/1 -> Mux2/3
  dy [m/s]/1 -> Mux2/2
  dx [m/s]/1 -> Mux2/1
  z [m]/1 -> Mux4/3
  y [m]/1 -> Mux4/2
  x [m]/1 -> Mux4/1
  Ground1/1 -> mux3/2  "pitch"
  Y [rad]/1 -> mux3/3, Mux3/3  "yaw"
  Mux3/1 -> Mux6/2
  Transformation_BODY2GLOBAL/1 -> Discrete-Time Integrator/1, Mux5/2  "VelVEH wrt  GLOB"
  mux3/1 -> Transformation_BODY2GLOBAL/2
  Ground/1 -> mux3/1  "roll"
  Mux2/1 -> Mux1/2, Transformation_BODY2GLOBAL/1
  Discrete-Time Integrator/1 -> Mux5/1  "PosVEH wrt  GLOB"

== system PPS_Scenario_006_cs/BMW_X5_1/SELF_Demux/compas converter ==
  rotz [rad] : Inport
  cart2compas : Subsystem
  rad2deg : Gain  Gain=180/pi
  heading [deg] : Outport
  wires:
  cart2compas/1(heading [deg]) -> heading [deg]/1
  rotz [rad]/1 -> rad2deg/1
  rad2deg/1 -> cart2compas/1(Angle [deg])

== system PPS_Scenario_006_cs/BMW_X5_2/Dynamics_Empty/MuxState ==
  note: mode: Dynamics
  note: mode: Positioning
  note: mode: Dynamics
      | VelVEHICLE
      | wrt VEH
  note: AnglesVEHICLE
      | wrtGLOB
  note: For state mode 'Dynamic' positions
      | are not taken into account, as they
      | are computed by integrating velocity.
      | Click annotation for Help.
  x [m] : Inport  SampleTime=TimeStep
  y [m] : Inport  Port=2  SampleTime=TimeStep
  z [m] : Inport  Port=3  SampleTime=TimeStep
  dx [m/s] : Inport  Port=4  SampleTime=TimeStep
  dy [m/s] : Inport  Port=5  SampleTime=TimeStep
  dz [m/s] : Inport  Port=6  SampleTime=TimeStep
  R [rad] : Inport  Port=7  SampleTime=TimeStep
  P [rad] : Inport  Port=8  SampleTime=TimeStep
  Y [rad] : Inport  Port=9  SampleTime=TimeStep
  Constant : Constant  DisableCoverage=on  Value=positioningmode
  Discrete-Time Integrator : DiscreteIntegrator  SampleTime=TimeStep  ICPrevOutput=DiscIntNeverNeededParam  ICPrevScaledInput=DiscIntNeverNeededParam
  Ground : Ground
  Ground1 : Ground
  Mux1 : Mux  Inputs=[3 3]
  Mux2 : Mux  Inputs=3
  Mux3 : Mux  Inputs=3
  Mux4 : Mux  Inputs=3
  Mux5 : Mux  Inputs=[3 3]
  Mux6 : Mux  Inputs=[6 3]
  Switch : Switch  Threshold=0.5
  Transformation_BODY2GLOBAL : PreScanSimulinkLibrary/Simple_Vehicle_Dynamics/Chassis/MuxDynState/Transformation_BODY2GLOBAL  SystemSampleTime=-1
  mux3 : Mux  Inputs=3
  state : Outport
  wires:
  Constant/1 -> Switch/2
  Mux6/1 -> state/1
  Mux4/1 -> Mux1/1
  Mux5/1 -> Switch/3
  Mux1/1 -> Switch/1
  Switch/1 -> Mux6/1  "PosVeh wrt  GLOB"
  P [rad]/1 -> Mux3/2
  R [rad]/1 -> Mux3/1
  dz [m/s]/1 -> Mux2/3
  dy [m/s]/1 -> Mux2/2
  dx [m/s]/1 -> Mux2/1
  z [m]/1 -> Mux4/3
  y [m]/1 -> Mux4/2
  x [m]/1 -> Mux4/1
  Ground1/1 -> mux3/2  "pitch"
  Y [rad]/1 -> mux3/3, Mux3/3  "yaw"
  Mux3/1 -> Mux6/2
  Transformation_BODY2GLOBAL/1 -> Discrete-Time Integrator/1, Mux5/2  "VelVEH wrt  GLOB"
  mux3/1 -> Transformation_BODY2GLOBAL/2
  Ground/1 -> mux3/1  "roll"
  Mux2/1 -> Mux1/2, Transformation_BODY2GLOBAL/1
  Discrete-Time Integrator/1 -> Mux5/1  "PosVEH wrt  GLOB"

== system PPS_Scenario_006_cs/BMW_X5_2/SELF_Demux/compas converter ==
  rotz [rad] : Inport
  cart2compas : Subsystem
  rad2deg : Gain  Gain=180/pi
  heading [deg] : Outport
  wires:
  cart2compas/1(heading [deg]) -> heading [deg]/1
  rotz [rad]/1 -> rad2deg/1
  rad2deg/1 -> cart2compas/1(Angle [deg])

== system PPS_Scenario_006_cs/BMW_Z3_1/Dynamics_Empty/MuxState ==
  note: mode: Dynamics
  note: mode: Positioning
  note: mode: Dynamics
      | VelVEHICLE
      | wrt VEH
  note: AnglesVEHICLE
      | wrtGLOB
  note: For state mode 'Dynamic' positions
      | are not taken into account, as they
      | are computed by integrating velocity.
      | Click annotation for Help.
  x [m] : Inport  SampleTime=TimeStep
  y [m] : Inport  Port=2  SampleTime=TimeStep
  z [m] : Inport  Port=3  SampleTime=TimeStep
  dx [m/s] : Inport  Port=4  SampleTime=TimeStep
  dy [m/s] : Inport  Port=5  SampleTime=TimeStep
  dz [m/s] : Inport  Port=6  SampleTime=TimeStep
  R [rad] : Inport  Port=7  SampleTime=TimeStep
  P [rad] : Inport  Port=8  SampleTime=TimeStep
  Y [rad] : Inport  Port=9  SampleTime=TimeStep
  Constant : Constant  DisableCoverage=on  Value=positioningmode
  Discrete-Time Integrator : DiscreteIntegrator  SampleTime=TimeStep  ICPrevOutput=DiscIntNeverNeededParam  ICPrevScaledInput=DiscIntNeverNeededParam
  Ground : Ground
  Ground1 : Ground
  Mux1 : Mux  Inputs=[3 3]
  Mux2 : Mux  Inputs=3
  Mux3 : Mux  Inputs=3
  Mux4 : Mux  Inputs=3
  Mux5 : Mux  Inputs=[3 3]
  Mux6 : Mux  Inputs=[6 3]
  Switch : Switch  Threshold=0.5
  Transformation_BODY2GLOBAL : PreScanSimulinkLibrary/Simple_Vehicle_Dynamics/Chassis/MuxDynState/Transformation_BODY2GLOBAL  SystemSampleTime=-1
  mux3 : Mux  Inputs=3
  state : Outport
  wires:
  Constant/1 -> Switch/2
  Mux6/1 -> state/1
  Mux4/1 -> Mux1/1
  Mux5/1 -> Switch/3
  Mux1/1 -> Switch/1
  Switch/1 -> Mux6/1  "PosVeh wrt  GLOB"
  P [rad]/1 -> Mux3/2
  R [rad]/1 -> Mux3/1
  dz [m/s]/1 -> Mux2/3
  dy [m/s]/1 -> Mux2/2
  dx [m/s]/1 -> Mux2/1
  z [m]/1 -> Mux4/3
  y [m]/1 -> Mux4/2
  x [m]/1 -> Mux4/1
  Ground1/1 -> mux3/2  "pitch"
  Y [rad]/1 -> mux3/3, Mux3/3  "yaw"
  Mux3/1 -> Mux6/2
  Transformation_BODY2GLOBAL/1 -> Discrete-Time Integrator/1, Mux5/2  "VelVEH wrt  GLOB"
  mux3/1 -> Transformation_BODY2GLOBAL/2
  Ground/1 -> mux3/1  "roll"
  Mux2/1 -> Mux1/2, Transformation_BODY2GLOBAL/1
  Discrete-Time Integrator/1 -> Mux5/1  "PosVEH wrt  GLOB"

== system PPS_Scenario_006_cs/BMW_Z3_1/SELF_Demux/compas converter ==
  rotz [rad] : Inport
  cart2compas : Subsystem
  rad2deg : Gain  Gain=180/pi
  heading [deg] : Outport
  wires:
  cart2compas/1(heading [deg]) -> heading [deg]/1
  rotz [rad]/1 -> rad2deg/1
  rad2deg/1 -> cart2compas/1(Angle [deg])

== system PPS_Scenario_006_cs/CarTrailer_SingleAxle_1/SELF_Demux/compas converter ==
  rotz [rad] : Inport
  cart2compas : Subsystem
  rad2deg : Gain  Gain=180/pi
  heading [deg] : Outport
  wires:
  cart2compas/1(heading [deg]) -> heading [deg]/1
  rotz [rad]/1 -> rad2deg/1
  rad2deg/1 -> cart2compas/1(Angle [deg])

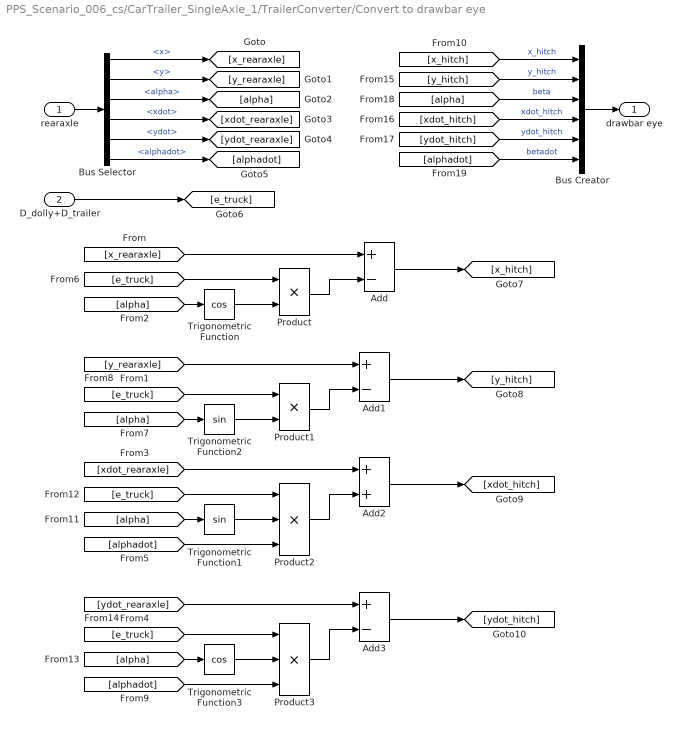
== system PPS_Scenario_006_cs/CarTrailer_SingleAxle_1/TrailerConverter/Convert to drawbar eye ==
  rearaxle : Inport
  D_dolly+D_trailer : Inport  Port=2
  Add : Sum  Inputs=+-
  Add1 : Sum  Inputs=+-
  Add2 : Sum
  Add3 : Sum  Inputs=+-
  Bus Creator : BusCreator  Inputs=6
  Bus Selector : BusSelector  OutputSignals=x,y,alpha,xdot,ydot,alphadot
  Product : Product  RndMeth=Zero
  Product1 : Product  RndMeth=Zero
  Product2 : Product  Inputs=3  RndMeth=Zero
  Product3 : Product  Inputs=3  RndMeth=Zero
  Trigonometric Function : Trigonometry  Operator=cos
  Trigonometric Function1 : Trigonometry
  Trigonometric Function2 : Trigonometry
  Trigonometric Function3 : Trigonometry  Operator=cos
  drawbar eye : Outport
  wires:
  Bus Creator/1 -> drawbar eye/1
  [alphadot] -> Bus Creator/6  "betadot"
  [ydot_hitch] -> Bus Creator/5  "ydot_hitch"
  [xdot_hitch] -> Bus Creator/4  "xdot_hitch"
  [alpha] -> Bus Creator/3  "beta"
  [y_hitch] -> Bus Creator/2  "y_hitch"
  [x_hitch] -> Bus Creator/1  "x_hitch"
  [alphadot] -> Product3/3
  [alphadot] -> Product2/3
  [alpha] -> Trigonometric Function3/1
  Trigonometric Function3/1 -> Product3/2
  Product3/1 -> Add3/2
  [e_truck] -> Product2/1
  [alpha] -> Trigonometric Function1/1
  Trigonometric Function1/1 -> Product2/2
  Product2/1 -> Add2/2
  Add3/1 -> [ydot_hitch]
  [ydot_rearaxle] -> Add3/1
  [e_truck] -> Product3/1
  Add2/1 -> [xdot_hitch]
  [xdot_rearaxle] -> Add2/1
  [alpha] -> Trigonometric Function2/1
  Trigonometric Function2/1 -> Product1/2
  Product1/1 -> Add1/2
  [e_truck] -> Product/1
  [alpha] -> Trigonometric Function/1
  Trigonometric Function/1 -> Product/2
  Product/1 -> Add/2
  Add1/1 -> [y_hitch]
  [y_rearaxle] -> Add1/1
  [e_truck] -> Product1/1
  Add/1 -> [x_hitch]
  [x_rearaxle] -> Add/1
  D_dolly+D_trailer/1 -> [e_truck]
  Bus Selector/6 -> [alphadot]  "<alphadot>"
  Bus Selector/5 -> [ydot_rearaxle]  "<ydot>"
  Bus Selector/4 -> [xdot_rearaxle]  "<xdot>"
  Bus Selector/3 -> [alpha]  "<alpha>"
  Bus Selector/2 -> [y_rearaxle]  "<y>"
  Bus Selector/1 -> [x_rearaxle]  "<x>"
  rearaxle/1 -> Bus Selector/1

== system PPS_Scenario_006_cs/CarTrailer_SingleAxle_1/TrailerConverter/Traj2State2 ==
  TrailerTraj : Inport
  Traj2State2 : Subsystem
  state : Outport
  wires:
  TrailerTraj/1 -> Traj2State2/1(traj)
  Traj2State2/1(state) -> state/1

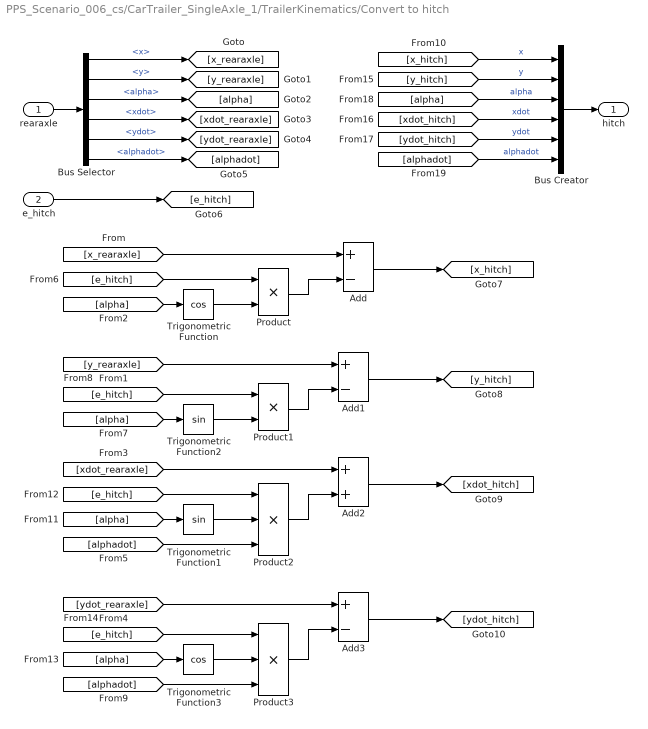
== system PPS_Scenario_006_cs/CarTrailer_SingleAxle_1/TrailerKinematics/Convert to hitch ==
  rearaxle : Inport
  e_hitch : Inport  Port=2
  Add : Sum  Inputs=+-
  Add1 : Sum  Inputs=+-
  Add2 : Sum
  Add3 : Sum  Inputs=+-
  Bus Creator : BusCreator  Inputs=6
  Bus Selector : BusSelector  OutputSignals=x,y,alpha,xdot,ydot,alphadot
  Product : Product  RndMeth=Zero
  Product1 : Product  RndMeth=Zero
  Product2 : Product  Inputs=3  RndMeth=Zero
  Product3 : Product  Inputs=3  RndMeth=Zero
  Trigonometric Function : Trigonometry  Operator=cos
  Trigonometric Function1 : Trigonometry
  Trigonometric Function2 : Trigonometry
  Trigonometric Function3 : Trigonometry  Operator=cos
  hitch : Outport
  wires:
  rearaxle/1 -> Bus Selector/1
  Bus Selector/1 -> [x_rearaxle]  "<x>"
  Bus Selector/2 -> [y_rearaxle]  "<y>"
  Bus Selector/3 -> [alpha]  "<alpha>"
  Bus Selector/4 -> [xdot_rearaxle]  "<xdot>"
  Bus Selector/5 -> [ydot_rearaxle]  "<ydot>"
  Bus Selector/6 -> [alphadot]  "<alphadot>"
  e_hitch/1 -> [e_hitch]
  [x_rearaxle] -> Add/1
  Add/1 -> [x_hitch]
  [e_hitch] -> Product1/1
  [y_rearaxle] -> Add1/1
  Add1/1 -> [y_hitch]
  Product/1 -> Add/2
  Trigonometric Function/1 -> Product/2
  [alpha] -> Trigonometric Function/1
  [e_hitch] -> Product/1
  Product1/1 -> Add1/2
  Trigonometric Function2/1 -> Product1/2
  [alpha] -> Trigonometric Function2/1
  [xdot_rearaxle] -> Add2/1
  Add2/1 -> [xdot_hitch]
  [e_hitch] -> Product3/1
  [ydot_rearaxle] -> Add3/1
  Add3/1 -> [ydot_hitch]
  Product2/1 -> Add2/2
  Trigonometric Function1/1 -> Product2/2
  [alpha] -> Trigonometric Function1/1
  [e_hitch] -> Product2/1
  Product3/1 -> Add3/2
  Trigonometric Function3/1 -> Product3/2
  [alpha] -> Trigonometric Function3/1
  [alphadot] -> Product2/3
  [alphadot] -> Product3/3
  [x_hitch] -> Bus Creator/1  "x"
  [y_hitch] -> Bus Creator/2  "y"
  [alpha] -> Bus Creator/3  "alpha"
  [xdot_hitch] -> Bus Creator/4  "xdot"
  [ydot_hitch] -> Bus Creator/5  "ydot"
  [alphadot] -> Bus Creator/6  "alphadot"
  Bus Creator/1 -> hitch/1

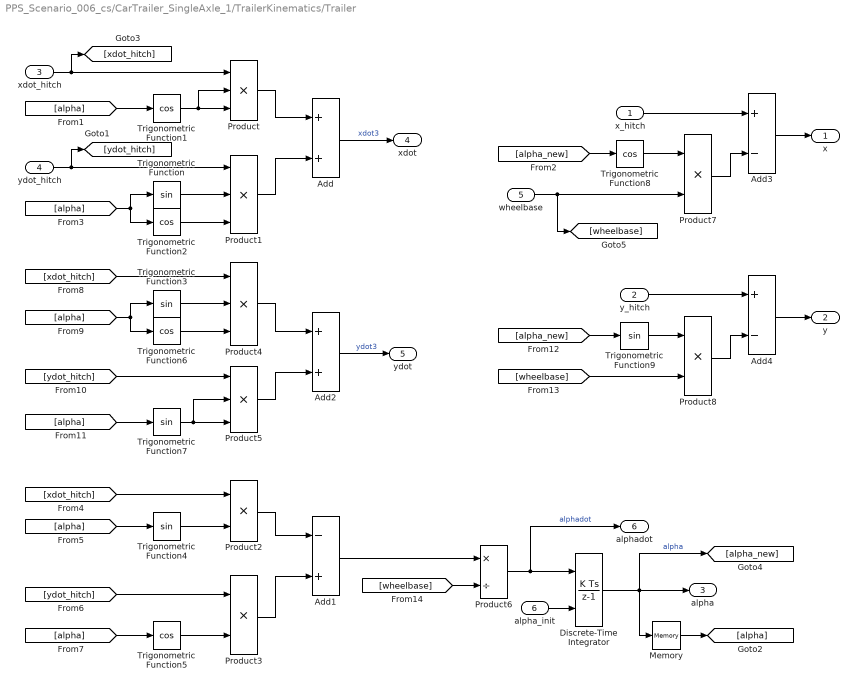
== system PPS_Scenario_006_cs/CarTrailer_SingleAxle_1/TrailerKinematics/Trailer ==
  x_hitch : Inport
  y_hitch : Inport  Port=2
  xdot_hitch : Inport  Port=3
  ydot_hitch : Inport  Port=4
  wheelbase : Inport  Port=5
  alpha_init : Inport  Port=6
  Add : Sum
  Add1 : Sum  Inputs=-+
  Add2 : Sum
  Add3 : Sum  Inputs=+-
  Add4 : Sum  Inputs=+-
  Discrete-Time Integrator : DiscreteIntegrator  InitialConditionSource=external  SampleTime=TimeStep  ICPrevOutput=DiscIntNeverNeededParam  ICPrevScaledInput=DiscIntNeverNeededParam
  Memory : Memory
  Product{,1,4..5} (4 alike) : Product  Inputs=3  RndMeth=Zero
  Product{2..3,7..8} (4 alike) : Product  RndMeth=Zero
  Product6 : Product  Inputs=*/  RndMeth=Zero
  Trigonometric Function{,3..4,7,9} (5 alike) : Trigonometry
  Trigonometric Function{1..2,5..6,8} (5 alike) : Trigonometry  Operator=cos
  x : Outport
  y : Outport  Port=2
  alpha : Outport  Port=3
  xdot : Outport  Port=4
  ydot : Outport  Port=5
  alphadot : Outport  Port=6
  wires:
  Trigonometric Function1/1 -> Product/3, Product/2
  Product/1 -> Add/1
  ydot_hitch/1 -> Product1/1, [ydot_hitch]
  Trigonometric Function2/1 -> Product1/3
  Product1/1 -> Add/2
  Trigonometric Function/1 -> Product1/2
  [alpha] -> Trigonometric Function2/1, Trigonometric Function/1
  Add/1 -> xdot/1  "xdot3"
  [alpha] -> Trigonometric Function4/1
  [xdot_hitch] -> Product2/1
  Trigonometric Function4/1 -> Product2/2
  Product2/1 -> Add1/1
  [ydot_hitch] -> Product3/1
  Trigonometric Function5/1 -> Product3/2
  Product3/1 -> Add1/2
  [alpha] -> Trigonometric Function5/1
  [xdot_hitch] -> Product4/1
  Trigonometric Function6/1 -> Product4/3
  Product4/1 -> Add2/1
  [ydot_hitch] -> Product5/1
  Trigonometric Function7/1 -> Product5/3, Product5/2
  Product5/1 -> Add2/2
  [alpha] -> Trigonometric Function7/1
  Add2/1 -> ydot/1  "ydot3"
  Trigonometric Function3/1 -> Product4/2
  [alpha] -> Trigonometric Function3/1, Trigonometric Function6/1
  Add1/1 -> Product6/1
  [wheelbase] -> Product6/2
  Product6/1 -> Discrete-Time Integrator/1, alphadot/1  "alphadot"
  alpha_init/1 -> Discrete-Time Integrator/2
  Discrete-Time Integrator/1 -> Memory/1, alpha/1, [alpha_new]  "alpha"
  xdot_hitch/1 -> Product/1, [xdot_hitch]
  [alpha] -> Trigonometric Function1/1
  [alpha_new] -> Trigonometric Function8/1
  Add3/1 -> x/1
  x_hitch/1 -> Add3/1
  [alpha_new] -> Trigonometric Function9/1
  Add4/1 -> y/1
  y_hitch/1 -> Add4/1
  Product8/1 -> Add4/2
  [wheelbase] -> Product8/2
  Trigonometric Function9/1 -> Product8/1
  Product7/1 -> Add3/2
  wheelbase/1 -> Product7/2, [wheelbase]
  Trigonometric Function8/1 -> Product7/1
  Memory/1 -> [alpha]

== system PPS_Scenario_006_cs/Child_RegularAni_1/SELF_Demux/compas converter ==
  rotz [rad] : Inport
  cart2compas : Subsystem
  rad2deg : Gain  Gain=180/pi
  heading [deg] : Outport
  wires:
  cart2compas/1(heading [deg]) -> heading [deg]/1
  rotz [rad]/1 -> rad2deg/1
  rad2deg/1 -> cart2compas/1(Angle [deg])

== system PPS_Scenario_006_cs/Child_RegularAni_1/Trajectories/Traj2State1 ==
  Traj Org : Inport
  Offset : Inport  Port=2
  Add2 : Sum
  ApplyRotation : PreScanSimulinkLibrary/ApplyRotation  SystemSampleTime=-1
  ApplyRotation1 : PreScanSimulinkLibrary/ApplyRotation  SystemSampleTime=-1
  ApplyRotation2 : PreScanSimulinkLibrary/ApplyRotation  SystemSampleTime=-1
  Constant : Constant  Value=zeros(12,1)
  Mux : Mux  Inputs=6
  Mux1 : Mux  Inputs=2
  Mux{2,4..9} (7 alike) : Mux  Inputs=3
  Mux3 : Mux  Inputs=2
  Selector : Selector  InputPortWidth=6  IndexOptions=Index vector (dialog)  Indices=[4 5 6]  OutputSizes=1
  Selector1 : Selector  InputPortWidth=21  IndexOptions=Index vector (dialog)  Indices=[5]  OutputSizes=1
  Selector10 : Selector  InputPortWidth=21  IndexOptions=Index vector (dialog)  Indices=[2]  OutputSizes=1
  Selector11 : Selector  InputPortWidth=21  IndexOptions=Index vector (dialog)  Indices=[3]  OutputSizes=1
  Selector12 : Selector  InputPortWidth=21  IndexOptions=Index vector (dialog)  Indices=[1]  OutputSizes=1
  Selector13 : Selector  InputPortWidth=21  IndexOptions=Index vector (dialog)  Indices=[8]  OutputSizes=1
  Selector14 : Selector  InputPortWidth=21  IndexOptions=Index vector (dialog)  Indices=[9]  OutputSizes=1
  Selector15 : Selector  InputPortWidth=21  IndexOptions=Index vector (dialog)  Indices=[7]  OutputSizes=1
  Selector16 : Selector  InputPortWidth=21  IndexOptions=Index vector (dialog)  Indices=[14]  OutputSizes=1
  Selector17 : Selector  InputPortWidth=21  IndexOptions=Index vector (dialog)  Indices=[15]  OutputSizes=1
  Selector18 : Selector  InputPortWidth=21  IndexOptions=Index vector (dialog)  Indices=[13]  OutputSizes=1
  Selector19 : Selector  InputPortWidth=21  IndexOptions=Index vector (dialog)  Indices=[20]  OutputSizes=1
  Selector2 : Selector  InputPortWidth=21  IndexOptions=Index vector (dialog)  Indices=[6]  OutputSizes=1
  Selector20 : Selector  InputPortWidth=21  IndexOptions=Index vector (dialog)  Indices=[21]  OutputSizes=1
  Selector21 : Selector  InputPortWidth=21  IndexOptions=Index vector (dialog)  Indices=[19]  OutputSizes=1
  Selector3 : Selector  InputPortWidth=21  IndexOptions=Index vector (dialog)  Indices=[12]  OutputSizes=1
  Selector4 : Selector  InputPortWidth=21  IndexOptions=Index vector (dialog)  Indices=[17]  OutputSizes=1
  Selector5 : Selector  InputPortWidth=21  IndexOptions=Index vector (dialog)  Indices=[18]  OutputSizes=1
  Selector6 : Selector  InputPortWidth=21  IndexOptions=Index vector (dialog)  Indices=[16]  OutputSizes=1
  Selector7 : Selector  InputPortWidth=21  IndexOptions=Index vector (dialog)  Indices=[11]  OutputSizes=1
  Selector8 : Selector  InputPortWidth=21  IndexOptions=Index vector (dialog)  Indices=[10]  OutputSizes=1
  Selector9 : Selector  InputPortWidth=21  IndexOptions=Index vector (dialog)  Indices=[4]  OutputSizes=1
  Traj2State2 : Subsystem
  state : Outport
  wires:
  Mux9/1 -> ApplyRotation2/2, ApplyRotation1/2, ApplyRotation/2
  Selector20/1 -> Mux9/3
  Selector19/1 -> Mux9/2
  Selector21/1 -> Mux9/1
  Selector5/1 -> Mux8/3
  Selector4/1 -> Mux8/2
  Selector6/1 -> Mux8/1
  Mux8/1 -> Mux/6
  Mux6/1 -> ApplyRotation2/1
  Mux7/1 -> Mux/4
  ApplyRotation2/1 -> Mux/5
  Selector3/1 -> Mux7/3
  Selector7/1 -> Mux7/2
  Selector8/1 -> Mux7/1
  Mux4/1 -> Mux/2
  Mux5/1 -> ApplyRotation1/1
  ApplyRotation1/1 -> Mux/3
  Mux2/1 -> ApplyRotation/1
  ApplyRotation/1 -> Mux/1
  Selector2/1 -> Mux4/3
  Selector1/1 -> Mux4/2
  Selector9/1 -> Mux4/1
  Selector17/1 -> Mux6/3
  Selector16/1 -> Mux6/2
  Selector18/1 -> Mux6/1
  Selector14/1 -> Mux5/3
  Selector13/1 -> Mux5/2
  Selector15/1 -> Mux5/1
  Selector11/1 -> Mux2/3
  Selector10/1 -> Mux2/2
  Selector12/1 -> Mux2/1
  Mux3/1 -> Selector8/1, Selector7/1, Selector3/1, Selector18/1, Selector16/1, Selector17/1, Selector6/1, Selector20/1, Selector19/1, Selector21/1, Selector5/1, Selector4/1, Selector14/1, Selector13/1, Selector15/1, Selector2/1, Selector1/1, Selector9/1, Selector12/1, Selector10/1, Selector11/1
  Mux1/1 -> Add2/2
  Constant/1 -> Mux1/2
  Add2/1 -> Traj2State2/1(traj)
  Selector/1 -> Mux3/2
  Traj Org/1 -> Mux3/1
  Offset/1 -> Mux1/1, Selector/1
  Mux/1 -> Add2/1
  Traj2State2/1(state) -> state/1

== system PPS_Scenario_006_cs/Child_RegularAni_1/Trajectories/Trajectory_3 ==
  From Workspace : FromWorkspace  VariableName=trajectory  SampleTime=TimeStep  OutputAfterFinalValue=Holding final value
  From Workspace1 : FromWorkspace  VariableName=trajectory  SampleTime=TimeStep  OutputAfterFinalValue=Setting to zero
  Mux : Mux  Inputs=2
  Selector1 : Selector  InputPortWidth=24  IndexOptions=Index vector (dialog)  Indices=[7:18]  OutputSizes=1
  Selector9 : Selector  InputPortWidth=24  IndexOptions=Index vector (dialog)  Indices=[1:6]  OutputSizes=1
  trajectory : Outport
  wires:
  Selector1/1 -> Mux/2
  Selector9/1 -> Mux/1
  Mux/1 -> trajectory/1
  From Workspace1/1 -> Selector1/1
  From Workspace/1 -> Selector9/1

== system PPS_Scenario_006_cs/Fiat_Bravo_1/Dynamics_Empty/MuxState ==
  note: mode: Dynamics
  note: mode: Positioning
  note: mode: Dynamics
      | VelVEHICLE
      | wrt VEH
  note: AnglesVEHICLE
      | wrtGLOB
  note: For state mode 'Dynamic' positions
      | are not taken into account, as they
      | are computed by integrating velocity.
      | Click annotation for Help.
  x [m] : Inport  SampleTime=TimeStep
  y [m] : Inport  Port=2  SampleTime=TimeStep
  z [m] : Inport  Port=3  SampleTime=TimeStep
  dx [m/s] : Inport  Port=4  SampleTime=TimeStep
  dy [m/s] : Inport  Port=5  SampleTime=TimeStep
  dz [m/s] : Inport  Port=6  SampleTime=TimeStep
  R [rad] : Inport  Port=7  SampleTime=TimeStep
  P [rad] : Inport  Port=8  SampleTime=TimeStep
  Y [rad] : Inport  Port=9  SampleTime=TimeStep
  Constant : Constant  DisableCoverage=on  Value=positioningmode
  Discrete-Time Integrator : DiscreteIntegrator  SampleTime=TimeStep  ICPrevOutput=DiscIntNeverNeededParam  ICPrevScaledInput=DiscIntNeverNeededParam
  Ground : Ground
  Ground1 : Ground
  Mux1 : Mux  Inputs=[3 3]
  Mux2 : Mux  Inputs=3
  Mux3 : Mux  Inputs=3
  Mux4 : Mux  Inputs=3
  Mux5 : Mux  Inputs=[3 3]
  Mux6 : Mux  Inputs=[6 3]
  Switch : Switch  Threshold=0.5
  Transformation_BODY2GLOBAL : PreScanSimulinkLibrary/Simple_Vehicle_Dynamics/Chassis/MuxDynState/Transformation_BODY2GLOBAL  SystemSampleTime=-1
  mux3 : Mux  Inputs=3
  state : Outport
  wires:
  Constant/1 -> Switch/2
  Mux6/1 -> state/1
  Mux4/1 -> Mux1/1
  Mux5/1 -> Switch/3
  Mux1/1 -> Switch/1
  Switch/1 -> Mux6/1  "PosVeh wrt  GLOB"
  P [rad]/1 -> Mux3/2
  R [rad]/1 -> Mux3/1
  dz [m/s]/1 -> Mux2/3
  dy [m/s]/1 -> Mux2/2
  dx [m/s]/1 -> Mux2/1
  z [m]/1 -> Mux4/3
  y [m]/1 -> Mux4/2
  x [m]/1 -> Mux4/1
  Ground1/1 -> mux3/2  "pitch"
  Y [rad]/1 -> mux3/3, Mux3/3  "yaw"
  Mux3/1 -> Mux6/2
  Transformation_BODY2GLOBAL/1 -> Discrete-Time Integrator/1, Mux5/2  "VelVEH wrt  GLOB"
  mux3/1 -> Transformation_BODY2GLOBAL/2
  Ground/1 -> mux3/1  "roll"
  Mux2/1 -> Mux1/2, Transformation_BODY2GLOBAL/1
  Discrete-Time Integrator/1 -> Mux5/1  "PosVEH wrt  GLOB"

== system PPS_Scenario_006_cs/Fiat_Bravo_1/SELF_Demux/compas converter ==
  rotz [rad] : Inport
  cart2compas : Subsystem
  rad2deg : Gain  Gain=180/pi
  heading [deg] : Outport
  wires:
  cart2compas/1(heading [deg]) -> heading [deg]/1
  rotz [rad]/1 -> rad2deg/1
  rad2deg/1 -> cart2compas/1(Angle [deg])
